simulink model "four_states_sym"  (R2013a)
settings: Solver=ode45  StartTime=0.0  StopTime=10.0  RelTol=1e-3
settings Model: Creator=Sunil  LastModifiedBy=Sunil

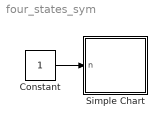
== system four_states_sym ==
  Constant : Constant
  Simple Chart : Stateflow chart  TreatAsAtomicUnit=on
  wires:
  Constant/1 -> Simple Chart/1(n)

== stateflow chart four_states_sym/Simple Chart ==
  state A
    en: x = x + 2;
    y = y + 1;
    du:
    ex:
  note: []/{}
  state start
    en: x = n;
    y = 1;
    du:
    ex:
  state C
    en:
    du:
    ex: y = y + 5;
  state end
    en:
    du:
    ex:
  state B
    en: x = x - 1;
    y = y - 1;
    du:
    ex:
  A -> C [order 2] : [x~=10]/{update()}
  C -> A [order 1] : [x < 10]/{update()}
  (default) -> start : {init()}
  A -> end [order 1] : [x == 10]/{update()}
  start -> C : []/{update()}
  C -> B [order 2] : []/{update()}
  B -> end [order 1] : [x==10]/{update()}
  B -> C [order 2] : [x~=10]/{update()}
  data: n input; x local double; y local double
  function init:
    | function init
    |     coder.extrinsic('run');
    |     run initEnv
  function update:
    | function update
    |   coder.extrinsic('run');
    |   run updateEnv;
